simulink model "lab_part1"  (R2022a)
settings: Solver=ode45  StartTime=0.0  StopTime=3  MaxStep=0.001  RelTol=1e-3
values from neighbouring files (symbols this model uses):
  A = [-6, -25; 1, 0]    [part3_plot.m]
  B = [25;0]    [part3_plot.m]
  C = [1,0;0,1]    [part3_plot.m]
  D = [0;0]    [part3_plot.m]
settings Model: Creator=zhong  LastModifiedBy=zhong
settings DataIOCC: LimitDataPoints=on

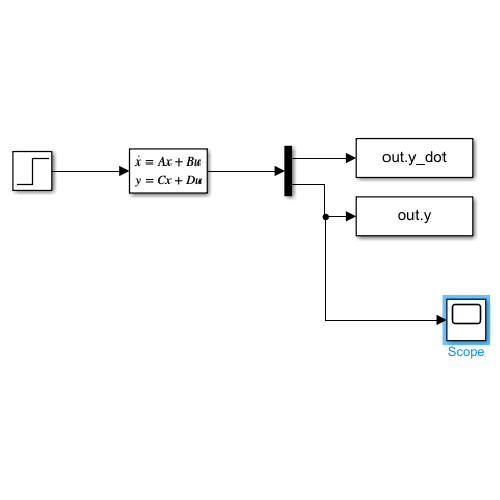
[thumbnail: Simulink's stored preview of the top-level diagram]
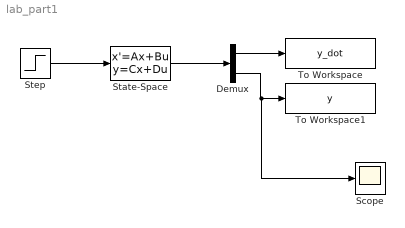
== system lab_part1 ==
  Demux : Demux  Outputs=2
  Scope : Scope
  State-Space : StateSpace  A=A  B=B  C=C  D=D  InitialCondition=0
  Step : Step  Time=0  SampleTime=0
  To Workspace : ToWorkspace  VariableName=y_dot  SampleTime=-1
  To Workspace1 : ToWorkspace  VariableName=y  SaveFormat=Structure With Time  SampleTime=-1
  wires:
  Step/1 -> State-Space/1
  State-Space/1 -> Demux/1
  Demux/1 -> To Workspace/1
  Demux/2 -> Scope/1, To Workspace1/1
